simulink model "edge"  (Simulink 8.3)
settings: Solver=ode45  StartTime=0.0  StopTime=10.0  RelTol=1e-3
settings Model: Creator=elkhadiy  LastModifiedBy=elkhadiy
settings DataIOCC: SignalLoggingSaveFormat=Dataset
settings DebuggingCC: UnderspecifiedInitializationDetection=Simplified  StateNameClashWarn=none
settings GRTTargetCC: CombineOutputUpdateFcns=on  GRTInterface=off

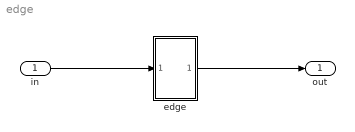
== system edge ==
  in : Inport  OutDataTypeStr=boolean
  edge : Subsystem
  out : Outport  OutDataTypeStr=boolean
  wires:
  in/1 -> edge/1(In1)
  edge/1(Out1) -> out/1

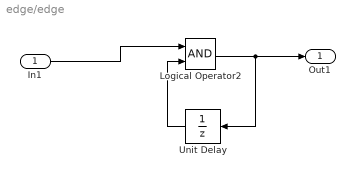
== system edge/edge ==
  In1 : Inport
  Logical Operator2 : Logic  AllPortsSameDT=off  OutDataTypeStr=boolean
  Unit Delay : UnitDelay  SampleTime=-1
  Out1 : Outport
  wires:
  In1/1 -> Logical Operator2/1
  Logical Operator2/1 -> Out1/1, Unit Delay/1
  Unit Delay/1 -> Logical Operator2/2
